simulink model "if_cond"  (R2021b)
settings: Solver=VariableStepAuto  StartTime=0.0  StopTime=10.0  RelTol=1e-3
undefined symbols (not defined in the file): DiscIntNeverNeededParam, Newton, Raphson
libraries: simulink x9, slpidlib x1
settings Model: NumberOfSteps=10  Creator=user  LastModifiedBy=cemery

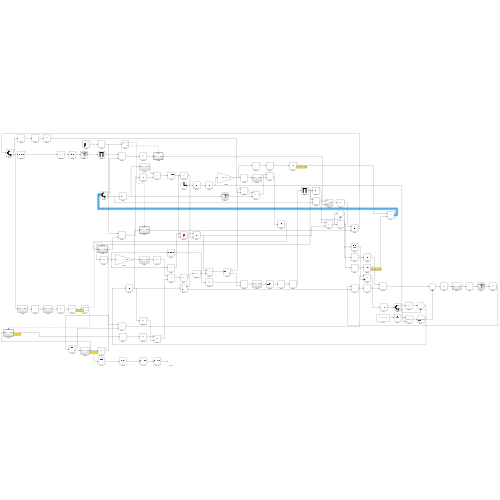
[thumbnail: Simulink's stored preview of the top-level diagram]
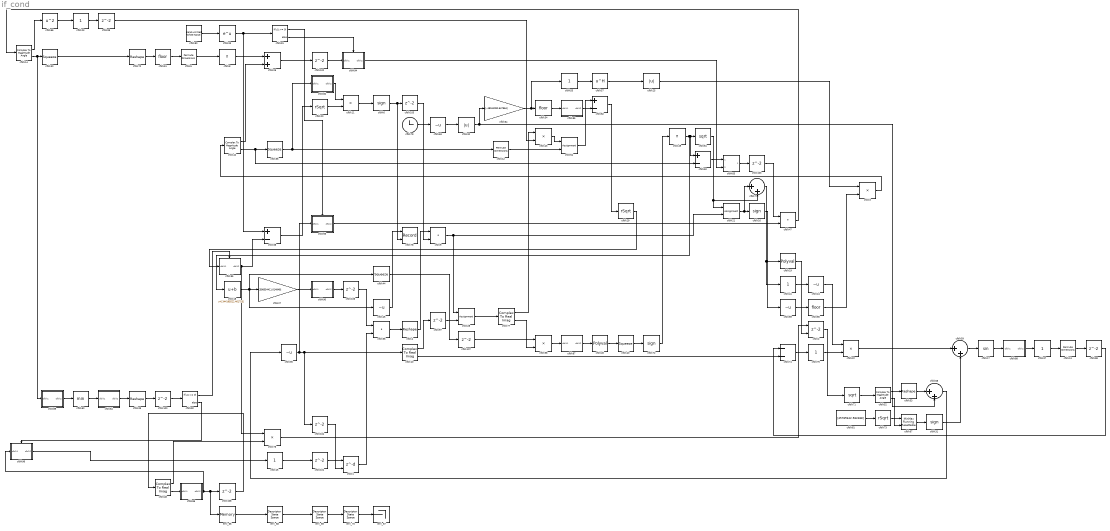
== system if_cond ==
  cfblk1 : Delay  DelayLengthSource=Input port  SampleTime=1
      settings: InputPortMap=u0,p1
  cfblk10 : ComplexToRealImag
  cfblk{97..108} (12 alike) : Delay  SampleTime=1
  cfblk11 : Product  Inputs=**
  cfblk12 : PermuteDimensions
  cfblk13 : PermuteDimensions
  cfblk14 : ComplexToMagnitudeAngle
  cfblk{15,23,37,41,55,75} (6 alike) : simulink/Math Operations/Slider Gain  gain=1  low=0  high=2
  cfblk{6,16,31,72} (4 alike) : Signum
  cfblk17 : Trigonometry
  cfblk18 : Bias  Bias=[344195522.461753]
  cfblk19 : Polyval  Coefs=[ +2.081618890e-019, -1.441693666e-014, +4.719686976e-010, -8.536869453e-006, +1.621573104e-001, -8.087801117e+001 ]
  cfblk2 : Delay  ShowEnablePort=on  SampleTime=1
      settings: InputPortMap=u0,e6
  cfblk20 : Sqrt  Operator=rSqrt  AlgorithmType=Newton-Raphson  SaturateOnIntegerOverflow=on
  cfblk21 : Assignment  DiagnosticForDimensions=Warning  IndexOptions=Index vector (dialog)  Indices=1  OutputSizes=1
  cfblk{3,22,58,76} (4 alike) : Product
  cfblk{24,35,45,63,69} (5 alike) : UnaryMinus
  cfblk25 : Abs
  cfblk26 : Sum
  cfblk27 : Gain  Gain=[398554411.014848]
  cfblk28 : Assignment  DiagnosticForDimensions=Warning  IndexOptions=Index vector (dialog)  Indices=1  OutputSizes=1
  cfblk29 : Sqrt  Operator=rSqrt  AlgorithmType=Newton-Raphson  SaturateOnIntegerOverflow=on
  cfblk{30,36,40,44} (4 alike) : Squeeze
  cfblk32 : Abs
  cfblk33 : Math  SaturateOnIntegerOverflow=on
  cfblk34 : Rounding
  cfblk38 : Sum  Inputs=+-
  cfblk{4,39,53,70} (4 alike) : Reshape
  cfblk42 : ComplexToMagnitudeAngle
  cfblk43 : Product  Inputs=**
  cfblk46 : Polyval  Coefs=[ +2.081618890e-019, -1.441693666e-014, +4.719686976e-010, -8.536869453e-006, +1.621573104e-001, -8.087801117e+001 ]
  cfblk47 : DotProduct  InputSameDT=on  OutDataTypeStr=Inherit: Inherit via internal rule
  cfblk48 : ComplexToRealImag
  cfblk49 : Product  Inputs=*
  cfblk5 : PermuteDimensions
  cfblk50 : Sum  Inputs=+-
  cfblk51 : Rounding
  cfblk52 : ComplexToMagnitudeAngle
  cfblk54 : Assignment  DiagnosticForDimensions=Warning  IndexOptions=Index vector (dialog)  Indices=1  OutputSizes=1
  cfblk56 : DotProduct  InputSameDT=on  OutDataTypeStr=Inherit: Inherit via internal rule
  cfblk57 : Math  Operator=hermitian  SaturateOnIntegerOverflow=on
  cfblk59 : Sum  Inputs=|++
  cfblk60 : MinMax
  cfblk61 : Sqrt  SaturateOnIntegerOverflow=on
  cfblk62 : Sum  Inputs=+-
  cfblk64 : Gain  Gain=[-48161092.647964]
  cfblk65 : Rounding
  cfblk66 : Math  Operator=square  SaturateOnIntegerOverflow=on
  cfblk67 : simulink/Math Operations/MinMax Running Resettable  Function=min  vinit=0.0
  cfblk68 : Sum  Inputs=|++
  cfblk7 : Sum  Inputs=|++
  cfblk71 : Sqrt  SaturateOnIntegerOverflow=on
  cfblk73 : Sqrt  Operator=rSqrt  AlgorithmType=Newton-Raphson  SaturateOnIntegerOverflow=on
  cfblk74 : Sum  Inputs=--
  cfblk77 : ComplexToRealImag
  cfblk78 : Record  FileSettingsInternal="{\"entries\":[{\"content\":{\"excelSettings\":{\"content\":{},\"type\":\"Streamout.ExcelSettings\"}},\"type\":\"Streamout.FileSettingStorage\",\"uuid\":\"ac85a95f-4be8-4778-839d-d844e6bad3ff\"}],\"packageUris\":[\"http://schema.mathworks.com/mf0/streamout_blocks/R2020a\"],\"version\":\"1.0\"}"  Layout=[1 1]  SignalsInternal="{\"entries\":[{\"content\":{\"signals\":[{\"content\":{\"blockPath\":[\"sampleModel400_pp_1568_1_difftest/cfblk78\"],\"channel\":[],\"dimensions\":[1],\"domain\":\"sampleModel400_pp_1568_1_difftest/cfblk78\",\"lineColor\":\"#ff6929\",\"plots\":[],\"port\":1,\"sid\":[\"\"],\"signalID\":66299,\"signalName\":\"cfblk45\"},\"type\":\"RecordBlkView.Signal\",\"uuid\":\"a7a329db-ddd2-4490-90a3-0e073e7fe2cc\"},{\"content\":{\"blockPath\":[\"sampleModel400_pp_1568_1_difftest/cfblk78\"],\"channel\":[],\"dimensions\":[1],\"domain\":\"sampleModel400_pp_1568_1_difftest/cfblk78\",\"lineColor\":\"#b746ff\",\"plots\":[],\"port\":2,\"sid\":[\"\"],\"signalID\":66303,\"signalName\":\"cfblk6\"},\"type\":\"RecordBlkView.Signal\",\"uuid\":\"1f2b0494-88a5-4856-9598-5e9e1808c606\"}]},\"type\":\"RecordBlkView.InputSignals\",\"uuid\":\"762c1f52-65dc-4b2a-80eb-8e18fd0fa685\"}],\"packageUris\":[\"http://schema.mathworks.com/mf0/streamout_blocks/R2020a\"],\"version\":\"1.0\"}"  VisualizationBindings="{\"xyplotplugin\":{\"info\":[{\"series\":[],\"subplotID\":1}]}}"  CompatibilityTag=XY
  cfblk79 : Clock
  cfblk8 : Product  Inputs=*
  cfblk80 : simulink/Sources/Band-Limited White Noise  Cov=[5230539780.965611]  Ts=0.1  seed=[7656552899.000000]
  cfblk81 : Constant  Value=[45789342.582488]  SampleTime=1
  cfblk82 : Subsystem
  cfblk83 : Subsystem
  cfblk84 : Subsystem
  cfblk85 : Subsystem
  cfblk86 : Subsystem
  cfblk87 : Subsystem
  cfblk88 : Subsystem
  cfblk89 : Subsystem
  cfblk9 : DotProduct  InputSameDT=on  OutDataTypeStr=Inherit: Inherit via internal rule
  cfblk90 : Subsystem
  cfblk91 : If  IfExpression=u1 >= 0  SampleTime=1
  cfblk92 : If  IfExpression=u1 >= 0  SampleTime=1
  cfblk93 : Subsystem  TreatAsAtomicUnit=on
  cfblk94 : Subsystem  TreatAsAtomicUnit=on
  cfblk95 : Subsystem  TreatAsAtomicUnit=on
  cfblk96 : Subsystem  TreatAsAtomicUnit=on
  emi_66 : Memory
  emi_67 : Terminator
  emi_68 : DescriptorStateSpace
  emi_69 : DescriptorStateSpace
  emi_70 : DescriptorStateSpace
  wires:
  cfblk96/1(cfblk2) -> cfblk15/1
  cfblk44/1 -> cfblk107/1
  emi_69/1 -> emi_70/1
  cfblk10/2 -> cfblk74/2
  emi_70/1 -> emi_67/1
  cfblk108/1 -> cfblk48/1
  emi_66/1 -> emi_68/1
  emi_68/1 -> emi_69/1
  cfblk107/1 -> cfblk58/1
  cfblk100/1 -> cfblk92/1
  cfblk106/1 -> cfblk56/1
  cfblk10/1 -> cfblk97/1
  cfblk90/1(cfblk2) -> cfblk106/1
  cfblk81/1 -> cfblk73/1
  cfblk53/1 -> cfblk68/1
  cfblk105/1 -> cfblk9/2
  cfblk104/1 -> cfblk1/2
  cfblk68/1 -> cfblk35/1
  cfblk13/1 -> cfblk98/1
  cfblk103/1 -> cfblk47/1
  cfblk83/1(cfblk2) -> cfblk103/1
  cfblk102/1 -> cfblk94/1(cfblk1)
  cfblk26/1 -> cfblk102/1
  cfblk101/1 -> cfblk1/1
  cfblk15/1 -> cfblk101/1
  cfblk39/1 -> cfblk100/1
  cfblk99/1 -> cfblk43/2
  cfblk23/1 -> cfblk99/1
  cfblk98/1 -> cfblk74/1
  cfblk97/1 -> cfblk28/2
  cfblk92/2 -> cfblk96/Action
  cfblk4/1 -> cfblk9/1
  cfblk92/1 -> cfblk95/Action
  cfblk55/1 -> cfblk57/1
  cfblk91/2 -> cfblk94/Action
  cfblk91/1 -> cfblk93/Action
  cfblk48/2 -> cfblk86/1(cfblk1)
  cfblk70/1 -> cfblk51/1
  cfblk84/1(cfblk2) -> cfblk39/1
  cfblk63/1 -> cfblk32/1
  cfblk22/1 -> cfblk59/1
  cfblk72/1 -> cfblk49/1
  cfblk40/1 -> cfblk72/1
  cfblk12/1 -> cfblk54/2
  cfblk62/1 -> cfblk29/1
  cfblk94/1(cfblk2) -> cfblk83/2(cfblk4)
  cfblk57/1 -> cfblk25/1
  cfblk75/1 -> cfblk22/2
  cfblk65/1 -> cfblk3/2
  cfblk28/1 -> cfblk77/1
  cfblk85/1(cfblk2) -> cfblk62/2
  cfblk48/1 -> cfblk76/2
  cfblk52/2 -> cfblk67/2
  cfblk31/1 -> cfblk59/2
  cfblk54/1 -> cfblk62/1
  cfblk66/1 -> cfblk23/1
  cfblk2/1 -> cfblk71/1
  cfblk52/1 -> cfblk53/1
  cfblk56/1 -> cfblk4/1
  cfblk1/1 -> cfblk56/2
  cfblk59/1 -> cfblk17/1
  cfblk29/1 -> cfblk95/1(cfblk1)
  cfblk60/1 -> cfblk84/1(cfblk1)
  cfblk19/1 -> cfblk2/2
  cfblk38/1 -> cfblk20/1
  cfblk25/1 -> cfblk3/1
  cfblk77/2 -> cfblk58/2
  cfblk45/1 -> cfblk78/1
  cfblk34/1 -> cfblk85/1(cfblk1)
  cfblk76/1 -> cfblk2/1
  cfblk89/1(cfblk2) -> cfblk60/1
  cfblk69/1 -> cfblk65/1
  cfblk30/1 -> cfblk70/1
  cfblk14/1 -> cfblk66/1
  cfblk46/1 -> cfblk40/1
  cfblk42/1 -> cfblk26/2
  cfblk3/1 -> cfblk42/1
  cfblk74/1 -> cfblk75/1
  cfblk71/1 -> cfblk52/1
  cfblk20/1 -> cfblk11/2
  cfblk88/1(cfblk2) -> cfblk37/1
  cfblk80/1 -> cfblk33/1
  cfblk17/1 -> cfblk88/1(cfblk1)
  cfblk11/1 -> cfblk6/1
  cfblk24/1 -> cfblk22/1
  cfblk43/1 -> cfblk54/1
  cfblk41/1 -> cfblk24/1
  cfblk67/1 -> cfblk31/1
  cfblk51/1 -> cfblk5/1
  cfblk77/1 -> cfblk43/1
  cfblk73/1 -> cfblk67/1
  cfblk27/1 -> cfblk90/1(cfblk1)
  cfblk50/1 -> cfblk83/1(cfblk1)
  cfblk16/1 -> cfblk69/1
  cfblk37/1 -> cfblk13/1
  cfblk93/1(cfblk2) -> cfblk47/2
  cfblk47/1 -> cfblk14/1
  cfblk79/1 -> cfblk63/1
  cfblk82/1(cfblk2) -> cfblk11/1
  cfblk8/1 -> cfblk26/1
  cfblk87/1(cfblk2) -> cfblk46/1
  cfblk58/1 -> cfblk87/1(cfblk1)
  cfblk5/1 -> cfblk8/1
  cfblk32/1 -> cfblk68/2, cfblk64/1
  cfblk42/2 -> cfblk36/1, cfblk50/2
  cfblk6/1 -> cfblk78/2, cfblk105/1
  cfblk33/1 -> cfblk91/1, cfblk38/1
  cfblk95/1(cfblk2) -> cfblk76/1, cfblk38/2
  cfblk14/2 -> cfblk89/1(cfblk1), cfblk30/1
  cfblk35/1 -> cfblk104/1, cfblk10/1, cfblk93/1(cfblk1)
  cfblk7/1 -> cfblk19/1, cfblk41/1
  cfblk18/1 -> cfblk45/1, cfblk44/1, cfblk27/1
  cfblk49/1 -> cfblk61/1, cfblk50/1, cfblk18/1
  cfblk61/1 -> cfblk7/2, cfblk21/1
  cfblk86/1(cfblk2) -> emi_66/1, cfblk108/1, cfblk96/1(cfblk1)
  cfblk36/1 -> cfblk82/1(cfblk1), cfblk12/1
  cfblk9/1 -> cfblk28/1, cfblk21/2
  cfblk21/1 -> cfblk7/1, cfblk16/1
  cfblk64/1 -> cfblk55/1, cfblk34/1

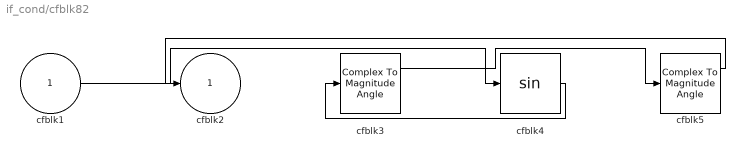
== system if_cond/cfblk82 ==
  cfblk1 : Inport
  cfblk3 : ComplexToMagnitudeAngle
  cfblk4 : Trigonometry
  cfblk5 : ComplexToMagnitudeAngle
  cfblk2 : Outport
  wires:
  cfblk1/1 -> cfblk4/1
  cfblk5/1 -> cfblk2/1
  cfblk4/1 -> cfblk3/1
  cfblk3/1 -> cfblk5/1

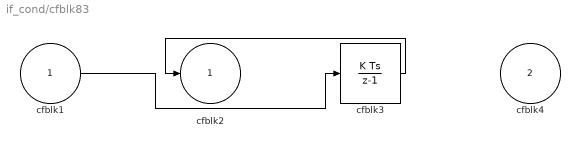
== system if_cond/cfblk83 ==
  cfblk1 : Inport
  cfblk4 : Inport  Port=2
  cfblk3 : DiscreteIntegrator  ICPrevOutput=DiscIntNeverNeededParam  ICPrevScaledInput=DiscIntNeverNeededParam
  cfblk2 : Outport
  wires:
  cfblk3/1 -> cfblk2/1
  cfblk1/1 -> cfblk3/1

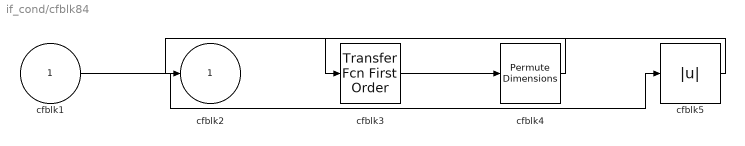
== system if_cond/cfblk84 ==
  cfblk1 : Inport
  cfblk3 : simulink/Discrete/Transfer Fcn First Order  PoleZ=0.95  ICPrevOutput=0.0  DoSatur=off
  cfblk4 : PermuteDimensions
  cfblk5 : Abs
  cfblk2 : Outport
  wires:
  cfblk5/1 -> cfblk3/1
  cfblk1/1 -> cfblk5/1
  cfblk4/1 -> cfblk2/1
  cfblk3/1 -> cfblk4/1

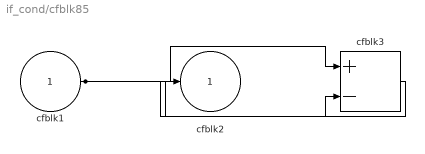
== system if_cond/cfblk85 ==
  cfblk1 : Inport
  cfblk3 : Sum  Inputs=+-
  cfblk2 : Outport
  wires:
  cfblk1/1 -> cfblk3/1, cfblk3/2
  cfblk3/1 -> cfblk2/1

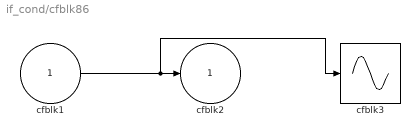
== system if_cond/cfblk86 ==
  cfblk1 : Inport
  cfblk3 : Sin  TimeSource=Use external signal  SampleTime=0
  cfblk2 : Outport
  wires:
  cfblk1/1 -> cfblk2/1, cfblk3/1

== system if_cond/cfblk87 ==
  cfblk1 : Inport
  cfblk3 : PermuteDimensions
  cfblk2 : Outport
  wires:
  cfblk1/1 -> cfblk2/1, cfblk3/1

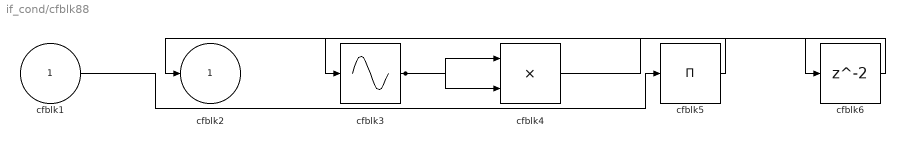
== system if_cond/cfblk88 ==
  cfblk1 : Inport
  cfblk3 : Sin  TimeSource=Use external signal  SampleTime=0
  cfblk4 : Product  Inputs=**
  cfblk5 : Product  Inputs=*
  cfblk6 : Delay  SampleTime=1
  cfblk2 : Outport
  wires:
  cfblk5/1 -> cfblk2/1
  cfblk1/1 -> cfblk5/1
  cfblk3/1 -> cfblk4/1, cfblk4/2
  cfblk4/1 -> cfblk6/1
  cfblk6/1 -> cfblk3/1

== system if_cond/cfblk89 ==
  cfblk1 : Inport
  cfblk3 : ComplexToRealImag
  cfblk2 : Outport
  wires:
  cfblk1/1 -> cfblk2/1, cfblk3/1

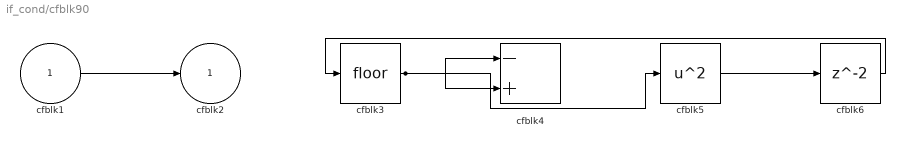
== system if_cond/cfblk90 ==
  cfblk1 : Inport
  cfblk3 : Rounding
  cfblk4 : Sum  Inputs=-+
  cfblk5 : Math  Operator=square  SaturateOnIntegerOverflow=on
  cfblk6 : Delay  SampleTime=1
  cfblk2 : Outport
  wires:
  cfblk3/1 -> cfblk5/1, cfblk4/1, cfblk4/2
  cfblk1/1 -> cfblk2/1
  cfblk5/1 -> cfblk6/1
  cfblk6/1 -> cfblk3/1

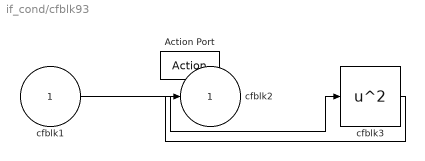
== system if_cond/cfblk93 ==
  cfblk1 : Inport
  Action Port : ActionPort  ActionPortLabel=if(u1 >= 0)
  cfblk3 : Math  Operator=square  SaturateOnIntegerOverflow=on
  cfblk2 : Outport
  wires:
  cfblk1/1 -> cfblk3/1
  cfblk3/1 -> cfblk2/1

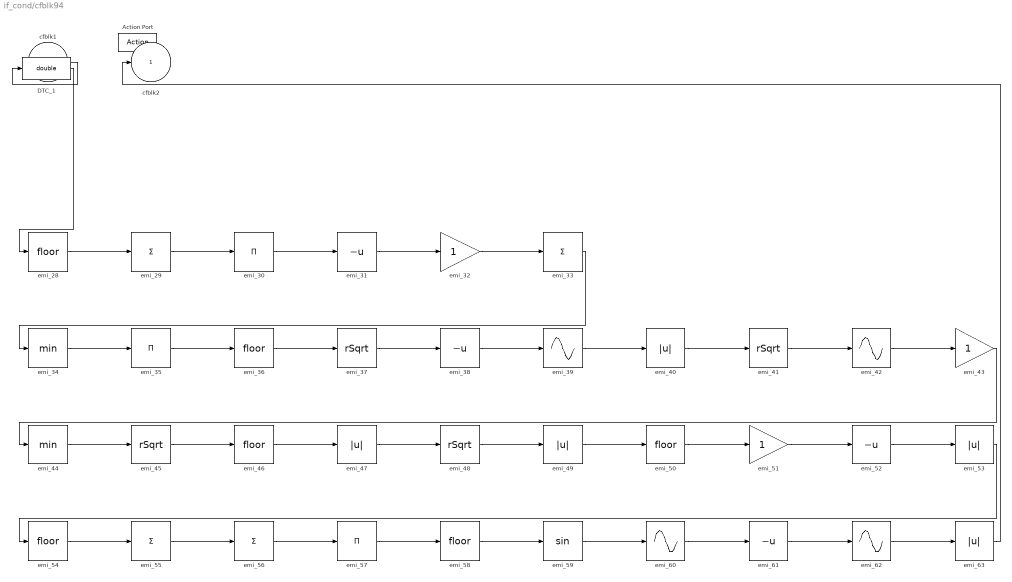
== system if_cond/cfblk94 ==
  cfblk1 : Inport
  Action Port : ActionPort  ActionPortLabel=else
  DTC_1 : DataTypeConversion  OutDataTypeStr=double
  emi_{28,36,46,50,54,58} (6 alike) : Rounding
  emi_{29,33,55..56} (4 alike) : Sum  Inputs=+
  emi_30 : Product  Inputs=*
  emi_{31,38,52,61} (4 alike) : UnaryMinus
  emi_32 : Gain
  emi_34 : MinMax
  emi_35 : Product  Inputs=*
  emi_{37,41,45,48} (4 alike) : Sqrt  Operator=rSqrt  SaturateOnIntegerOverflow=on
  emi_{39,42,60,62} (4 alike) : Sin  TimeSource=Use external signal  SampleTime=0
  emi_{40,47,49,53,63} (5 alike) : Abs
  emi_43 : Gain
  emi_44 : MinMax
  emi_51 : Gain
  emi_57 : Product  Inputs=*
  emi_59 : Trigonometry
  cfblk2 : Outport
  wires:
  cfblk1/1 -> DTC_1/1
  DTC_1/1 -> emi_28/1
  emi_28/1 -> emi_29/1
  emi_29/1 -> emi_30/1
  emi_30/1 -> emi_31/1
  emi_31/1 -> emi_32/1
  emi_32/1 -> emi_33/1
  emi_33/1 -> emi_34/1
  emi_34/1 -> emi_35/1
  emi_35/1 -> emi_36/1
  emi_36/1 -> emi_37/1
  emi_37/1 -> emi_38/1
  emi_38/1 -> emi_39/1
  emi_39/1 -> emi_40/1
  emi_40/1 -> emi_41/1
  emi_41/1 -> emi_42/1
  emi_42/1 -> emi_43/1
  emi_43/1 -> emi_44/1
  emi_44/1 -> emi_45/1
  emi_45/1 -> emi_46/1
  emi_46/1 -> emi_47/1
  emi_47/1 -> emi_48/1
  emi_48/1 -> emi_49/1
  emi_49/1 -> emi_50/1
  emi_50/1 -> emi_51/1
  emi_51/1 -> emi_52/1
  emi_52/1 -> emi_53/1
  emi_53/1 -> emi_54/1
  emi_54/1 -> emi_55/1
  emi_55/1 -> emi_56/1
  emi_56/1 -> emi_57/1
  emi_57/1 -> emi_58/1
  emi_58/1 -> emi_59/1
  emi_59/1 -> emi_60/1
  emi_60/1 -> emi_61/1
  emi_61/1 -> emi_62/1
  emi_62/1 -> emi_63/1
  emi_63/1 -> cfblk2/1

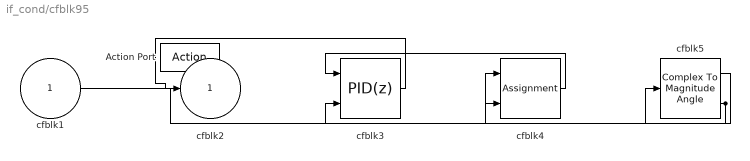
== system if_cond/cfblk95 ==
  cfblk1 : Inport
  Action Port : ActionPort  ActionPortLabel=if(u1 >= 0)
  cfblk3 : slpidlib/PID Controller (2DOF)  Controller=PID  Form=Parallel  TimeDomain=Discrete-time  UseExternalTs=off  SampleTime=-1  IntegratorMethod=Forward Euler  FilterMethod=Forward Euler  ControllerParametersSource=internal  P=1  I=1  D=0  UseFilter=on  N=100  b=1  c=1  TunerSelectOption=Transfer Function Based (PID Tuner App)  InitialConditionSource=internal  InitialConditionForIntegrator=0  InitialConditionForFilter=0  DifferentiatorICPrevScaledInput=0  ExternalReset=none  TrackingMode=off  Kt=1  LimitOutput=off  SatLimitsSource=internal  UpperSaturationLimit=inf  LowerSaturationLimit=-inf  LinearizeAsGain=off  AntiWindupMode=none  Kb=1  POutMin=[]  POutMax=[]  IOutMin=[]  IOutMax=[]  DOutMin=[]  DOutMax=[]  NOutMin=[]  NOutMax=[]  bOutMin=[]  bOutMax=[]  cOutMin=[]  cOutMax=[]  SumOutMin=[]  SumOutMax=[]  SaturationOutMin=[]  SaturationOutMax=[]  PParamMin=[]  PParamMax=[]  IParamMin=[]  IParamMax=[]  DParamMin=[]  DParamMax=[]  NParamMin=[]  NParamMax=[]  bParamMin=[]  bParamMax=[]  cParamMin=[]  cParamMax=[]  KbParamMin=[]  KbParamMax=[]  KtParamMin=[]  KtParamMax=[]  KbOutMin=[]  KbOutMax=[]  KtOutMin=[]  KtOutMax=[]  IntegratorOutMin=[]  IntegratorOutMax=[]  FilterOutMin=[]  FilterOutMax=[]  SumI1OutMin=[]  SumI1OutMax=[]  SumI2OutMin=[]  SumI2OutMax=[]  SumI3OutMin=[]  SumI3OutMax=[]  SumI4OutMin=[]  SumI4OutMax=[]  SumDOutMin=[]  SumDOutMax=[]  Sum1OutMin=[]  Sum1OutMax=[]  Sum2OutMin=[]  Sum2OutMax=[]  Sum3OutMin=[]  Sum3OutMax=[]  DifferentiatorOutMin=[]  DifferentiatorOutMax=[]  FilterDiffOutCoefMin=[]  FilterDiffOutCoefMax=[]  ReciprocalOutMin=[]  ReciprocalOutMax=[]  SumDenOutMin=[]  SumDenOutMax=[]  SumNumOutMin=[]  SumNumOutMax=[]  DivideOutMin=[]  DivideOutMax=[]  UdiffTsProdOutMin=[]  UdiffTsProdOutMax=[]  NTsProdOutMin=[]  NTsProdOutMax=[]  UintegralTsProdOutMin=[]  UintegralTsProdOutMax=[]  UngainTsProdOutMin=[]  UngainTsProdOutMax=[]  IntegratorContinuousStateAttributes=''  IntegratorStateMustResolveToSignalObject=off  IntegratorRTWStateStorageClass=Auto  FilterContinuousStateAttributes=''  FilterStateMustResolveToSignalObject=off  FilterRTWStateStorageClass=Auto  ParallelPVariant=InternalParameters  IdealPVariant=Disabled  IVariant=InternalParameters  DVariant=InternalParameters  bVariant=InternalParameters  cVariant=InternalParameters  IntegratorVariant=Discrete  SatVariant=Disabled  AWVariant=Passthrough  PCopyVariant=Disabled  TRVariant=Disabled  FdbkBlocksVariant=Forward  IdealPFdbkVariant=Disabled  SatFdbkVariant=Disabled  DerivativeFilterVariant=ForwardEulerFilter  NVariant=InternalParameters  NCopyVariant=Disabled  FilterICVariant=InternalICsFilter  IntegratorICVariant=InternalICs  ExternalResetVariant=Disabled  TRSumVariant=Passthrough  SumFdbkVariant=Disabled  SumVariant=Sum_PID  TsampFilterVariant=InternalTs  TsampNgainVariant=Passthrough  TsampIntegralVariant=Passthrough  ExternalSaturationOutDataTypeStr=Inherit: Same as second input
      settings: SourceProductBaseCode=SL
  cfblk4 : Assignment  DiagnosticForDimensions=Warning  IndexOptions=Index vector (dialog)  Indices=1  OutputSizes=1
  cfblk5 : ComplexToMagnitudeAngle
  cfblk2 : Outport
  wires:
  cfblk1/1 -> cfblk5/1
  cfblk3/1 -> cfblk2/1
  cfblk4/1 -> cfblk3/1
  cfblk5/1 -> cfblk3/2
  cfblk5/2 -> cfblk4/1, cfblk4/2

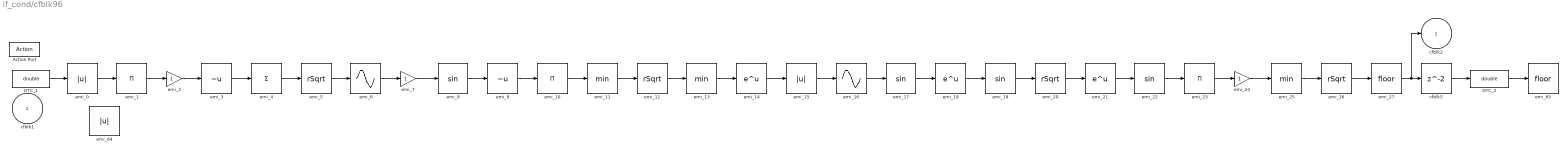
== system if_cond/cfblk96 ==
  cfblk1 : Inport
  Action Port : ActionPort  ActionPortLabel=else
  DTC_1 : DataTypeConversion  OutDataTypeStr=double
  DTC_2 : DataTypeConversion  OutDataTypeStr=double
  cfblk5 : Delay
  emi_0 : Abs
  emi_1 : Product  Inputs=*
  emi_10 : Product  Inputs=*
  emi_11 : MinMax
  emi_{5,12,20,26} (4 alike) : Sqrt  Operator=rSqrt  SaturateOnIntegerOverflow=on
  emi_13 : MinMax
  emi_14 : Math  SaturateOnIntegerOverflow=on
  emi_15 : Abs
  emi_16 : Sin  TimeSource=Use external signal  SampleTime=0
  emi_{8,17,19,22} (4 alike) : Trigonometry
  emi_18 : Math  SaturateOnIntegerOverflow=on
  emi_2 : Gain
  emi_21 : Math  SaturateOnIntegerOverflow=on
  emi_23 : Product  Inputs=*
  emi_24 : Gain
  emi_25 : MinMax
  emi_27 : Rounding
  emi_3 : UnaryMinus
  emi_4 : Sum  Inputs=+
  emi_6 : Sin  TimeSource=Use external signal  SampleTime=0
  emi_64 : Abs
  emi_65 : Rounding
  emi_7 : Gain
  emi_9 : UnaryMinus
  cfblk2 : Outport
  wires:
  emi_21/1 -> emi_22/1
  emi_23/1 -> emi_24/1
  emi_24/1 -> emi_25/1
  emi_17/1 -> emi_18/1
  DTC_2/1 -> emi_65/1
  emi_22/1 -> emi_23/1
  emi_25/1 -> emi_26/1
  emi_26/1 -> emi_27/1
  emi_3/1 -> emi_4/1
  cfblk5/1 -> DTC_2/1
  emi_20/1 -> emi_21/1
  emi_19/1 -> emi_20/1
  emi_18/1 -> emi_19/1
  emi_10/1 -> emi_11/1
  emi_16/1 -> emi_17/1
  emi_15/1 -> emi_16/1
  emi_14/1 -> emi_15/1
  emi_13/1 -> emi_14/1
  emi_12/1 -> emi_13/1
  emi_11/1 -> emi_12/1
  emi_9/1 -> emi_10/1
  emi_27/1 -> cfblk5/1, cfblk2/1
  emi_8/1 -> emi_9/1
  emi_7/1 -> emi_8/1
  emi_6/1 -> emi_7/1
  emi_5/1 -> emi_6/1
  emi_4/1 -> emi_5/1
  emi_2/1 -> emi_3/1
  emi_1/1 -> emi_2/1
  emi_0/1 -> emi_1/1
  DTC_1/1 -> emi_0/1
